simulink model "valdir_2015b"  (R2015b)
settings: Solver=ode45  StartTime=0.0  StopTime=0.5  RelTol=1e-3
values from neighbouring files (symbols this model uses):
  Ao = Ac'    [lista_2.m]    (also in lista_5.m; ss2obsercanon.m)
  Bo = Cc'    [lista_2.m]    (also in lista_5.m; ss2obsercanon.m)
  Co = Bc'    [lista_2.m]    (also in lista_5.m; ss2obsercanon.m)
  K = solve(B,k)    [ATV1_AB2_SC2.m]    (also in andre_q6.m = acker(Ap, Bp, -5); estabilidade.m = 0.01:0.001:0.0670; estabilidade_1.m = 0.0:0.001:0.0670; exemploTopEspecificacao.m = acker(A, B, [-5]))
  L = acker(Ao',Co',polos)'    [lista_5.m]
undefined symbols (not defined in the file or in its folder): Ac, Bc, Cc
settings Model: Creator=Lazaros  LastModifiedBy=valdir
settings DataIOCC: SaveFormat=Array
settings DebuggingCC: UnderspecifiedInitializationDetection=Classic  MergeDetectMultiDrivingBlocksExec=none  SolverPrmCheckMsg=warning  AllowSymbolicDim=on  StateNameClashWarn=warning
settings HardwareCC: ProdBitPerPointer=32  ProdLargestAtomicFloat=None  ProdIntDivRoundTo=Undefined  ProdEndianess=Unspecified  ProdWordSize=32  ProdHWDeviceType=32-bit Generic
settings GRTTargetCC: GeneratePreprocessorConditionals=Disable all
settings ConfigComp: CovModelRefEnable=Off

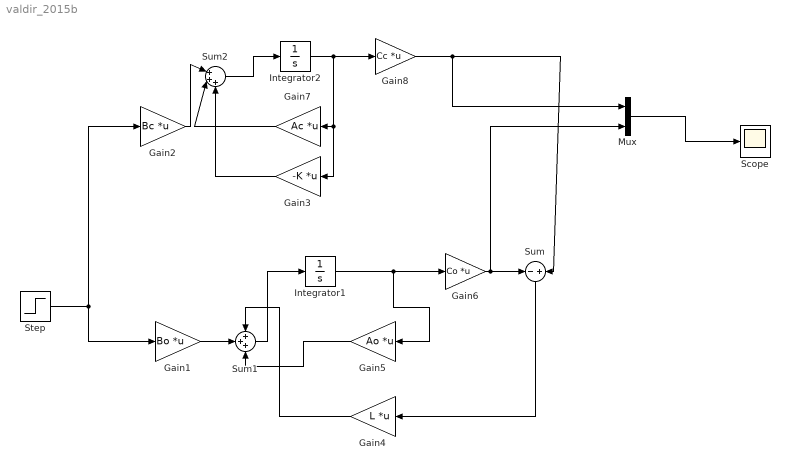
== system valdir_2015b ==
  Gain1 : Gain  Gain=Bo  Multiplication=Matrix(K*u)
  Gain2 : Gain  Gain=Bc  Multiplication=Matrix(K*u)
  Gain3 : Gain  Gain=-K  Multiplication=Matrix(K*u)
  Gain4 : Gain  Gain=L  Multiplication=Matrix(K*u)
  Gain5 : Gain  Gain=Ao  Multiplication=Matrix(K*u)
  Gain6 : Gain  Gain=Co  Multiplication=Matrix(K*u)
  Gain7 : Gain  Gain=Ac  Multiplication=Matrix(K*u)
  Gain8 : Gain  Gain=Cc  Multiplication=Matrix(K*u)
  Integrator1 : Integrator  InitialCondition=0.5
  Integrator2 : Integrator
  Mux : Mux  Inputs=2
  Scope : Scope
  Step : Step  SampleTime=0
  Sum : Sum  Inputs=-|+
  Sum1 : Sum  Inputs=+++
  Sum2 : Sum  Inputs=|+++
  wires:
  Integrator1/1 -> Gain5/1, Gain6/1
  Sum/1 -> Gain4/1
  Integrator2/1 -> Gain8/1, Gain3/1, Gain7/1
  Gain2/1 -> Sum2/1
  Gain7/1 -> Sum2/2
  Sum2/1 -> Integrator2/1
  Gain8/1 -> Mux/1, Sum/2
  Gain6/1 -> Mux/2, Sum/1
  Mux/1 -> Scope/1
  Gain3/1 -> Sum2/3
  Gain1/1 -> Sum1/2
  Gain5/1 -> Sum1/3
  Gain4/1 -> Sum1/1
  Sum1/1 -> Integrator1/1
  Step/1 -> Gain2/1, Gain1/1
